simulink model "manipulator_identification_q3"  (R2020a)
settings: Solver=VariableStepAuto  StartTime=0.0  StopTime=Ttot  RelTol=1e-3
undefined symbols (not defined in the file): dT_target, Fq_interp, KpPos_3, KpVel_3, Q_interp, Qp_interp, Qpp_interp, smiData, TdPos_3, TdVel_3, TiPos_3, TiVel_3, X, Y, Z
libraries: sm_lib x46, nesl_utility x23
(part 1 of 2)
settings Model: Creator=monti  LastModifiedBy=miche
settings DebuggingCC: SFMachineParentedDataDiag=error

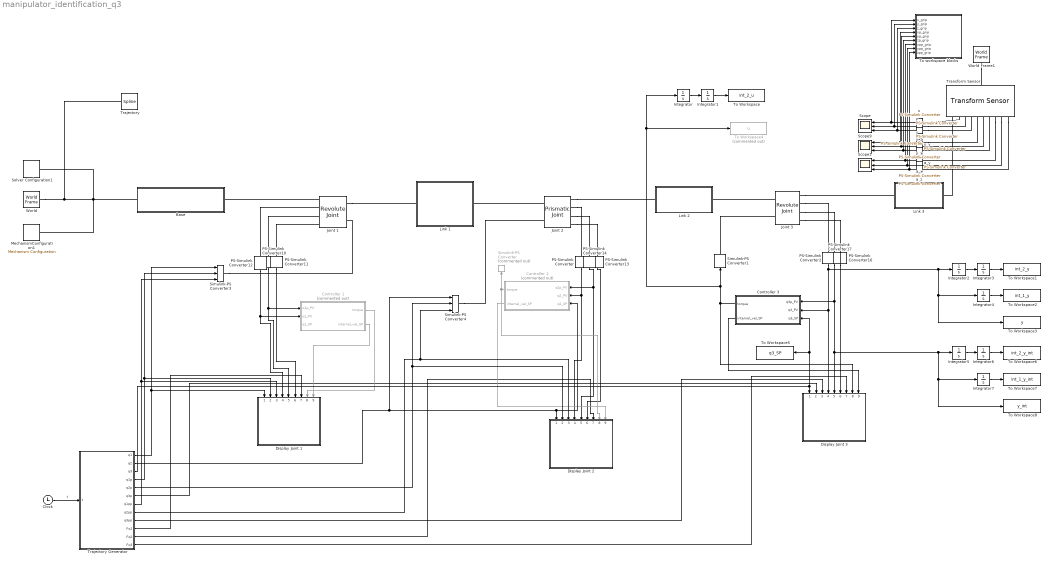
== system manipulator_identification_q3 ==
  Base : Subsystem
      mask Display: image('$imagefile'); % Use "Edit Image" on toolstrip to change.
  Clock : Clock
  Controller 1 : Subsystem  Commented=on
  Controller 2 : Subsystem  Commented=on
  Controller 3 : Subsystem
  Display Joint 1 : Subsystem
  Display Joint 2 : Subsystem
  Display Joint 3 : Subsystem
  Integrator{,1..7} (8 alike) : Integrator
  Joint 1 : sm_lib/Joints/Revolute Joint  JointMode=Normal  SenseConstraintForce=off  SenseConstraintForceX=off  SenseConstraintForceY=off  SenseConstraintForceZ=off  SenseConstraintTorque=off  SenseConstraintTorqueX=off  SenseConstraintTorqueY=off  SenseConstraintTorqueZ=off  SenseTotalForce=off  SenseTotalForceX=off  SenseTotalForceY=off  SenseTotalForceZ=off  SenseTotalTorque=off  SenseTotalTorqueX=off  SenseTotalTorqueY=off  SenseTotalTorqueZ=off  CompositeWrenchDir=FollowerOnBase  CompositeWrenchFrame=BaseFrame  EquilibriumPosition=0  EquilibriumPositionUnits=rad  SpringStiffness=0  SpringStiffnessUnits=N*m/rad  DampingCoefficient=0  DampingCoefficientUnits=N*m/(rad/s)  TorqueActuationMode=ComputedTorque  MotionActuationMode=InputMotion  SensePosition=on  SenseVelocity=on  SenseAcceleration=on  SenseTorqueForce=off  SenseLowerLimitTorqueForce=off  SenseUpperLimitTorqueForce=off  LowerLimitSpecify=on  LowerLimitBound=-180  LowerLimitBoundUnits=deg  LowerLimitStiffness=1e4  LowerLimitStiffnessUnits=N*m/deg  LowerLimitDamping=10  LowerLimitDampingUnits=N*m/(deg/s)  LowerLimitTransitionRegionWidth=0.1  LowerLimitTransitionRegionWidthUnits=deg  UpperLimitSpecify=on  UpperLimitBound=180  UpperLimitBoundUnits=deg  UpperLimitStiffness=1e4  UpperLimitStiffnessUnits=N*m/deg  UpperLimitDamping=10  UpperLimitDampingUnits=N*m/(deg/s)  UpperLimitTransitionRegionWidth=0.1  UpperLimitTransitionRegionWidthUnits=deg  PositionTargetSpecify=on  PositionTargetPriority=Low  PositionTargetValue=0  PositionTargetValueUnits=deg  VelocityTargetSpecify=off  VelocityTargetPriority=High  VelocityTargetValue=0  VelocityTargetValueUnits=deg/s
  Joint 2 : sm_lib/Joints/Prismatic Joint  JointMode=Normal  SenseConstraintForce=off  SenseConstraintForceX=off  SenseConstraintForceY=off  SenseConstraintForceZ=off  SenseConstraintTorque=off  SenseConstraintTorqueX=off  SenseConstraintTorqueY=off  SenseConstraintTorqueZ=off  SenseTotalForce=off  SenseTotalForceX=off  SenseTotalForceY=off  SenseTotalForceZ=off  SenseTotalTorque=off  SenseTotalTorqueX=off  SenseTotalTorqueY=off  SenseTotalTorqueZ=off  CompositeWrenchDir=FollowerOnBase  CompositeWrenchFrame=BaseFrame  EquilibriumPosition=0  EquilibriumPositionUnits=m  SpringStiffness=0  SpringStiffnessUnits=N/m  DampingCoefficient=0  DampingCoefficientUnits=N/(m/s)  TorqueActuationMode=ComputedTorque  MotionActuationMode=InputMotion  SensePosition=on  SenseVelocity=on  SenseAcceleration=on  SenseTorqueForce=off  SenseLowerLimitTorqueForce=off  SenseUpperLimitTorqueForce=off  LowerLimitSpecify=on  LowerLimitBound=0  LowerLimitBoundUnits=m  LowerLimitStiffness=1e6  LowerLimitStiffnessUnits=N/m  LowerLimitDamping=1e3  LowerLimitDampingUnits=N/(m/s)  LowerLimitTransitionRegionWidth=1e-4  LowerLimitTransitionRegionWidthUnits=m  UpperLimitSpecify=on  UpperLimitBound=0.4  UpperLimitBoundUnits=m  UpperLimitStiffness=1e6  UpperLimitStiffnessUnits=N/m  UpperLimitDamping=1e3  UpperLimitDampingUnits=N/(m/s)  UpperLimitTransitionRegionWidth=1e-4  UpperLimitTransitionRegionWidthUnits=m  PositionTargetSpecify=on  PositionTargetPriority=Low  PositionTargetValue=0.000  PositionTargetValueUnits=m  VelocityTargetSpecify=off  VelocityTargetPriority=High  VelocityTargetValue=0  VelocityTargetValueUnits=m/s
  Joint 3 : sm_lib/Joints/Revolute Joint  JointMode=Normal  SenseConstraintForce=off  SenseConstraintForceX=off  SenseConstraintForceY=off  SenseConstraintForceZ=off  SenseConstraintTorque=off  SenseConstraintTorqueX=off  SenseConstraintTorqueY=off  SenseConstraintTorqueZ=off  SenseTotalForce=off  SenseTotalForceX=off  SenseTotalForceY=off  SenseTotalForceZ=off  SenseTotalTorque=off  SenseTotalTorqueX=off  SenseTotalTorqueY=off  SenseTotalTorqueZ=off  CompositeWrenchDir=FollowerOnBase  CompositeWrenchFrame=BaseFrame  EquilibriumPosition=0  EquilibriumPositionUnits=rad  SpringStiffness=0  SpringStiffnessUnits=N*m/rad  DampingCoefficient=0  DampingCoefficientUnits=N*m/(rad/s)  TorqueActuationMode=InputTorque  MotionActuationMode=ComputedMotion  SensePosition=on  SenseVelocity=on  SenseAcceleration=on  SenseTorqueForce=off  SenseLowerLimitTorqueForce=off  SenseUpperLimitTorqueForce=off  LowerLimitSpecify=on  LowerLimitBound=-90  LowerLimitBoundUnits=deg  LowerLimitStiffness=1e4  LowerLimitStiffnessUnits=N*m/deg  LowerLimitDamping=10  LowerLimitDampingUnits=N*m/(deg/s)  LowerLimitTransitionRegionWidth=0.1  LowerLimitTransitionRegionWidthUnits=deg  UpperLimitSpecify=on  UpperLimitBound=90  UpperLimitBoundUnits=deg  UpperLimitStiffness=1e4  UpperLimitStiffnessUnits=N*m/deg  UpperLimitDamping=10  UpperLimitDampingUnits=N*m/(deg/s)  UpperLimitTransitionRegionWidth=0.1  UpperLimitTransitionRegionWidthUnits=deg  PositionTargetSpecify=on  PositionTargetPriority=Low  PositionTargetValue=0  PositionTargetValueUnits=deg  VelocityTargetSpecify=off  VelocityTargetPriority=High  VelocityTargetValue=0  VelocityTargetValueUnits=deg/s
  Link 1 : Subsystem
      mask Display: image('$imagefile'); % Use "Edit Image" on toolstrip to change.
  Link 2 : Subsystem
      mask Display: image('$imagefile'); % Use "Edit Image" on toolstrip to change.
  Link 3 : Subsystem
      mask Display: image('$imagefile'); % Use "Edit Image" on toolstrip to change.
  MechanismConfiguration1 : sm_lib/Utilities/Mechanism Configuration  UniformGravity=Constant  GravityVector=[0 0 -9.80665]  GravityUnits=m/s^2  LinearizationDelta=0.001
  PS-Simulink Converter : nesl_utility/PS-Simulink Converter  PhysicalDomain=network_engine_domain  SubClassName=ps_output  LeftPortType=input  RightPortType=output  PseudoPeriodic=off  Frequencies=[]  Unit=m  AffineConversion=off
      settings: SourceProductBaseCode=PW,SS
  PS-Simulink Converter10 : nesl_utility/PS-Simulink Converter  PhysicalDomain=network_engine_domain  SubClassName=ps_output  LeftPortType=input  RightPortType=output  PseudoPeriodic=off  Frequencies=[]  Unit=rad/s  AffineConversion=off
      settings: SourceProductBaseCode=PW,SS
  PS-Simulink Converter11 : nesl_utility/PS-Simulink Converter  PhysicalDomain=network_engine_domain  SubClassName=ps_output  LeftPortType=input  RightPortType=output  PseudoPeriodic=off  Frequencies=[]  Unit=rad/s^2  AffineConversion=off
      settings: SourceProductBaseCode=PW,SS
  PS-Simulink Converter12 : nesl_utility/PS-Simulink Converter  PhysicalDomain=network_engine_domain  SubClassName=ps_output  LeftPortType=input  RightPortType=output  PseudoPeriodic=off  Frequencies=[]  Unit=rad  AffineConversion=off
      settings: SourceProductBaseCode=PW,SS
  PS-Simulink Converter13 : nesl_utility/PS-Simulink Converter  PhysicalDomain=network_engine_domain  SubClassName=ps_output  LeftPortType=input  RightPortType=output  PseudoPeriodic=off  Frequencies=[]  Unit=m/s^2  AffineConversion=off
      settings: SourceProductBaseCode=PW,SS
  PS-Simulink Converter14 : nesl_utility/PS-Simulink Converter  PhysicalDomain=network_engine_domain  SubClassName=ps_output  LeftPortType=input  RightPortType=output  PseudoPeriodic=off  Frequencies=[]  Unit=m/s  AffineConversion=off
      settings: SourceProductBaseCode=PW,SS
  PS-Simulink Converter16 : nesl_utility/PS-Simulink Converter  PhysicalDomain=network_engine_domain  SubClassName=ps_output  LeftPortType=input  RightPortType=output  PseudoPeriodic=off  Frequencies=[]  Unit=rad/s^2  AffineConversion=off
      settings: SourceProductBaseCode=PW,SS
  PS-Simulink Converter17 : nesl_utility/PS-Simulink Converter  PhysicalDomain=network_engine_domain  SubClassName=ps_output  LeftPortType=input  RightPortType=output  PseudoPeriodic=off  Frequencies=[]  Unit=rad/s  AffineConversion=off
      settings: SourceProductBaseCode=PW,SS
  PS-Simulink Converter2 : nesl_utility/PS-Simulink Converter  PhysicalDomain=network_engine_domain  SubClassName=ps_output  LeftPortType=input  RightPortType=output  PseudoPeriodic=off  Frequencies=[]  Unit=rad  AffineConversion=off
      settings: SourceProductBaseCode=PW,SS
  Scope : Scope  NumInputPorts=3
  Scope1 : Scope  NumInputPorts=3
  Scope9 : Scope  NumInputPorts=3
  Simulink-PS Converter : nesl_utility/Simulink-PS Converter  Commented=on  PhysicalDomain=network_engine_domain  SubClassName=ps_input  LeftPortType=input  RightPortType=output  PseudoPeriodic=off  Frequencies=[]  NoiseDistribution=none  NoiseParameters=[]  Unit=N  AffineConversion=off  FilteringAndDerivatives=provide  SimscapeFilterOrder=1  InputFilterTimeConstant=0.001  UdotUserProvided=0
  Simulink-PS Converter1 : nesl_utility/Simulink-PS Converter  PhysicalDomain=network_engine_domain  SubClassName=ps_input  LeftPortType=input  RightPortType=output  PseudoPeriodic=off  Frequencies=[]  NoiseDistribution=none  NoiseParameters=[]  Unit=N*m  AffineConversion=off  FilteringAndDerivatives=provide  SimscapeFilterOrder=1  InputFilterTimeConstant=0.001  UdotUserProvided=0
  Simulink-PS Converter3 : nesl_utility/Simulink-PS Converter  PhysicalDomain=network_engine_domain  SubClassName=ps_input  LeftPortType=input  RightPortType=output  PseudoPeriodic=off  Frequencies=[]  NoiseDistribution=none  NoiseParameters=[]  Unit=rad  AffineConversion=off  FilteringAndDerivatives=provide  SimscapeFilterOrder=2  InputFilterTimeConstant=0.001  UdotUserProvided=2
      settings: SourceProductBaseCode=PW,SS
  Simulink-PS Converter4 : nesl_utility/Simulink-PS Converter  PhysicalDomain=network_engine_domain  SubClassName=ps_input  LeftPortType=input  RightPortType=output  PseudoPeriodic=off  Frequencies=[]  NoiseDistribution=none  NoiseParameters=[]  Unit=m  AffineConversion=off  FilteringAndDerivatives=provide  SimscapeFilterOrder=2  InputFilterTimeConstant=0.001  UdotUserProvided=2
      settings: SourceProductBaseCode=PW,SS
  Solver Configuration1 : nesl_utility/Solver Configuration  PhysicalDomain=network_engine_domain  SubClassName=solver  LeftPortType=input  RightPortType=generic  Tones=[]  Harmonics=[]  SimulateNoise=off  Profile=off  UseLocalSampling=off  EnableSwitchedLinearOptims=on  FrequencyDomain=off  UseCCode=off  RelTol=0.001  AbsTol=1e-06  MinStep=1e-09  ToWorkspace=off  RevertToSquareIcSolve=off  NumHomotopyIterations=100  PhasorMode=off  PhasorModeNumHarmonics=1  DoDC=off  ResidualTolerance=1e-09  UseLocalSolver=off  LocalSolverChoice=NE_BACKWARD_EULER_ADVANCER  LocalSolverSampleTime=0.001  DoFixedCost=off  MaxNonlinIter=3  MaxModeIter=2  LinearAlgebra=auto  EquationFormulation=NE_TIME_EF  DelaysMemoryBudget=1024  AutomaticFiltering=on  FilteringTimeConstant=0.001  PartitionStorageMethod=AS_NEEDED  PartitionMemoryBudget=1024  PartitionMethod=ROBUST
      settings: SourceProductBaseCode=PW,SS
  To Workspace : ToWorkspace  VariableName=int_2_u  SaveFormat=Timeseries  SampleTime=-1
  To Workspace1 : ToWorkspace  VariableName=int_2_y  SaveFormat=Timeseries  SampleTime=-1
  To Workspace2 : ToWorkspace  VariableName=int_1_y  SaveFormat=Timeseries  SampleTime=-1
  To Workspace3 : ToWorkspace  VariableName=y  SaveFormat=Timeseries  SampleTime=-1
  To Workspace4 : ToWorkspace  Commented=on  VariableName=u  SaveFormat=Timeseries  SampleTime=-1
  To Workspace5 : ToWorkspace  VariableName=q3_SP  SaveFormat=Timeseries  SampleTime=-1
  To Workspace6 : ToWorkspace  VariableName=int_2_y_int  SaveFormat=Timeseries  SampleTime=-1
  To Workspace7 : ToWorkspace  VariableName=int_1_y_int  SaveFormat=Timeseries  SampleTime=-1
  To Workspace8 : ToWorkspace  VariableName=y_int  SaveFormat=Timeseries  SampleTime=-1
  To workspace blocks : Subsystem
  Trajectory : sm_lib/Curves and Surfaces/Spline  GraphicAmbientColor=[0.15 0.15 0.15 1.0]  GraphicDiffuseColor=[0.0 0.0 0.0]  DataPoints=S(1:3,2:end-1)'  DataPointsUnits=m  GraphicEmissiveColor=[0.0 0.0 0.0 1.0]  EndConditionType=Natural  MarkerShape=Sphere  MarkerSize=10  GraphicType=FromGeometry  GraphicOpacity=1  GraphicShininess=75  GraphicSpecularColor=[0.5 0.5 0.5 1.0]  GraphicVisPropType=SimpleVisualProperties
  Trajectory Generator : MATLAB Function  TreatAsAtomicUnit=on
  Transform Sensor : sm_lib/Frames and Transforms/Transform Sensor  MeasurementFrame=World  SenseAngle=off  SenseAxis=off  SenseAngle1=off  SenseAngle2=off  SenseAngle3=off  SenseQ=off  SenseR=off  SenseOmegaX=off  SenseOmegaY=off  SenseOmegaZ=off  SenseOmega1=off  SenseOmega2=off  SenseOmega3=off  SenseQDot=off  SenseRDot=off  SenseAlphaX=off  SenseAlphaY=off  SenseAlphaZ=off  SenseAlpha1=off  SenseAlpha2=off  SenseAlpha3=off  SenseQDDot=off  SenseRDDot=off  SenseX=on  SenseY=on  SenseZ=on  SenseRad=off  SenseAzim=off  SenseDist=off  SenseInc=off  SenseXDot=on  SenseYDot=on  SenseZDot=on  SenseRadDot=off  SenseAzimDot=off  SenseDistDot=off  SenseIncDot=off  SenseXDDot=on  SenseYDDot=on  SenseZDDot=on  SenseRadDDot=off  SenseAzimDDot=off  SenseDistDDot=off  SenseIncDDot=off
  World : sm_lib/Frames and Transforms/World Frame
  World Frame1 : sm_lib/Frames and Transforms/World Frame
  a_x : nesl_utility/PS-Simulink Converter  PhysicalDomain=network_engine_domain  SubClassName=ps_output  LeftPortType=input  RightPortType=output  PseudoPeriodic=off  Frequencies=[]  Unit=m/s^2  AffineConversion=off
  a_y : nesl_utility/PS-Simulink Converter  PhysicalDomain=network_engine_domain  SubClassName=ps_output  LeftPortType=input  RightPortType=output  PseudoPeriodic=off  Frequencies=[]  Unit=m/s^2  AffineConversion=off
  a_z : nesl_utility/PS-Simulink Converter  PhysicalDomain=network_engine_domain  SubClassName=ps_output  LeftPortType=input  RightPortType=output  PseudoPeriodic=off  Frequencies=[]  Unit=m/s^2  AffineConversion=off
  v_x : nesl_utility/PS-Simulink Converter  PhysicalDomain=network_engine_domain  SubClassName=ps_output  LeftPortType=input  RightPortType=output  PseudoPeriodic=off  Frequencies=[]  Unit=m/s  AffineConversion=off
  v_y : nesl_utility/PS-Simulink Converter  PhysicalDomain=network_engine_domain  SubClassName=ps_output  LeftPortType=input  RightPortType=output  PseudoPeriodic=off  Frequencies=[]  Unit=m/s  AffineConversion=off
  v_z : nesl_utility/PS-Simulink Converter  PhysicalDomain=network_engine_domain  SubClassName=ps_output  LeftPortType=input  RightPortType=output  PseudoPeriodic=off  Frequencies=[]  Unit=m/s  AffineConversion=off
  x : nesl_utility/PS-Simulink Converter  PhysicalDomain=network_engine_domain  SubClassName=ps_output  LeftPortType=input  RightPortType=output  PseudoPeriodic=off  Frequencies=[]  Unit=m  AffineConversion=off
  y : nesl_utility/PS-Simulink Converter  PhysicalDomain=network_engine_domain  SubClassName=ps_output  LeftPortType=input  RightPortType=output  PseudoPeriodic=off  Frequencies=[]  Unit=m  AffineConversion=off
  z : nesl_utility/PS-Simulink Converter  PhysicalDomain=network_engine_domain  SubClassName=ps_output  LeftPortType=input  RightPortType=output  PseudoPeriodic=off  Frequencies=[]  Unit=m  AffineConversion=off
  wires:
  Trajectory Generator/9(q3pp) -> Display Joint 3/3(qpp_SP)
  a_y/1 -> Scope1/2, To workspace blocks/8(ypp_grip)
  Clock/1 -> Trajectory Generator/1(t)  "t"
  z/1 -> Scope/3, To workspace blocks/3(z_grip)
  v_y/1 -> Scope9/2, To workspace blocks/5(yp_grip)
  v_z/1 -> Scope9/3, To workspace blocks/6(zp_grip)
  Trajectory Generator/6(q3p) -> Display Joint 3/2(qp_SP)
  PS-Simulink Converter16/1 -> Display Joint 3/6(qpp_PV)
  PS-Simulink Converter12/1 -> Controller 1/2(q1_PV), Display Joint 1/4(q_PV)
  PS-Simulink Converter10/1 -> Controller 1/1(q1p_PV), Display Joint 1/5(qp_PV)
  Trajectory Generator/11(Fq2) -> Display Joint 2/7(torque_theoric)
  PS-Simulink Converter11/1 -> Display Joint 1/6(qpp_PV)
  PS-Simulink Converter/1 -> Display Joint 2/4(q_PV), Controller 2/2(q2_PV)
  Controller 3/2(internal_vel_SP) -> Display Joint 3/9(internal_vel_SP)
  Trajectory Generator/12(Fq3) -> Display Joint 3/7(torque_theoric)
  Trajectory Generator/7(q1pp) -> Simulink-PS Converter3/3, Display Joint 1/3(qpp_SP)
  a_z/1 -> Scope1/3, To workspace blocks/9(zpp_grip)
  PS-Simulink Converter14/1 -> Display Joint 2/5(qp_PV), Controller 2/1(q2p_PV)
  Trajectory Generator/4(q1p) -> Simulink-PS Converter3/2, Display Joint 1/2(qp_SP)
  x/1 -> Scope/1, To workspace blocks/1(x_grip)
  v_x/1 -> Scope9/1, To workspace blocks/4(xp_grip)
  y/1 -> Scope/2, To workspace blocks/2(y_grip)
  PS-Simulink Converter13/1 -> Display Joint 2/6(qpp_PV)
  a_x/1 -> Scope1/1, To workspace blocks/7(xpp_grip)
  Controller 1/1(torque) -> Display Joint 1/8(torque_actual)
  Controller 1/2(internal_vel_SP) -> Display Joint 1/9(internal_vel_SP)
  Trajectory Generator/10(Fq1) -> Display Joint 1/7(torque_theoric)
  Controller 2/1(torque) -> Display Joint 2/8(torque_actual), Simulink-PS Converter/1
  Controller 2/2(internal_vel_SP) -> Display Joint 2/9(internal_vel_SP)
  Integrator4/1 -> To Workspace2/1
  Integrator2/1 -> Integrator3/1
  Integrator3/1 -> To Workspace1/1
  PS-Simulink Converter2/1 -> To Workspace3/1, Integrator4/1, Integrator2/1, Display Joint 3/4(q_PV), Controller 3/2(q3_PV)
  Integrator/1 -> Integrator1/1
  Integrator1/1 -> To Workspace/1
  Controller 3/1(torque) -> Display Joint 3/8(torque_actual), To Workspace4/1, Integrator/1, Simulink-PS Converter1/1
  Trajectory Generator/1(q1) -> Simulink-PS Converter3/1, Display Joint 1/1(q_SP)
  Trajectory Generator/5(q2p) -> Simulink-PS Converter4/2, Display Joint 2/2(qp_SP)
  Trajectory Generator/8(q2pp) -> Simulink-PS Converter4/3, Display Joint 2/3(qpp_SP)
  Trajectory Generator/2(q2) -> Simulink-PS Converter4/1, Controller 2/3(q2_SP), Display Joint 2/1(q_SP)
  Trajectory Generator/3(q3) -> Display Joint 3/1(q_SP), To Workspace5/1, Controller 3/3(q3_SP)
  Integrator6/1 -> To Workspace6/1
  PS-Simulink Converter17/1 -> To Workspace8/1, Integrator7/1, Integrator5/1, Display Joint 3/5(qp_PV), Controller 3/1(q3p_PV)
  Integrator7/1 -> To Workspace7/1
  Integrator5/1 -> Integrator6/1
  connections:
  MechanismConfiguration1/RConn1 -- World/RConn1 -- Trajectory/LConn1 -- Solver Configuration1/RConn1 -- Base/LConn1
  v_z/LConn1 -- Transform Sensor/RConn7
  Joint 3/LConn1 -- Link 2/RConn1
  Joint 2/RConn1 -- Link 2/LConn1
  Joint 1/RConn2 -- PS-Simulink Converter12/LConn1
  Joint 2/RConn2 -- PS-Simulink Converter/LConn1
  Joint 3/RConn3 -- PS-Simulink Converter17/LConn1
  Joint 1/LConn1 -- Link 1/LConn1
  v_y/LConn1 -- Transform Sensor/RConn6
  v_x/LConn1 -- Transform Sensor/RConn5
  Joint 3/RConn4 -- PS-Simulink Converter16/LConn1
  World Frame1/RConn1 -- Transform Sensor/LConn1
  Transform Sensor/RConn8 -- a_x/LConn1
  Joint 3/LConn2 -- Simulink-PS Converter1/RConn1
  Joint 2/RConn3 -- PS-Simulink Converter14/LConn1
  Joint 1/RConn4 -- PS-Simulink Converter11/LConn1
  z/LConn1 -- Transform Sensor/RConn4
  Joint 2/RConn4 -- PS-Simulink Converter13/LConn1
  Transform Sensor/RConn9 -- a_y/LConn1
  Joint 1/RConn3 -- PS-Simulink Converter10/LConn1
  Joint 3/RConn1 -- Link 3/RConn1
  Joint 2/LConn1 -- Link 1/RConn1
  Joint 3/RConn2 -- PS-Simulink Converter2/LConn1
  y/LConn1 -- Transform Sensor/RConn3
  Transform Sensor/RConn10 -- a_z/LConn1
  Joint 1/RConn1 -- Base/RConn1
  x/LConn1 -- Transform Sensor/RConn2
  Transform Sensor/RConn1 -- Link 3/LConn1
  Simulink-PS Converter3/RConn1 -- Joint 1/LConn2
  Simulink-PS Converter4/RConn1 -- Joint 2/LConn2

== system manipulator_identification_q3/Base ==
  Transform : sm_lib/Frames and Transforms/Rigid Transform  TranslationMethod=Cartesian  TranslationStandardOffset=0  TranslationLengthUnit=mm  TranslationStandardAxis=+Z  TranslationCartesianOffset=smiData.RigidTransform(17).translation  TranslationROffset=0  TranslationROffsetUnits=m  TranslationZOffset=0  TranslationZOffsetUnits=m  TranslationThetaOffset=0  TranslationThetaOffsetUnits=deg  RotationMethod=ArbitraryAxis  RotationAngleUnits=rad  RotationStandardAxis=+Z  RotationAngle=smiData.RigidTransform(17).angle  RotationArbitraryAxis=smiData.RigidTransform(17).axis  FollAlignAxisA=+X  BaseAlignAxisA=+Y  FollAlignAxisB=+Y  BaseAlignAxisB=+Z  RotationSequenceAxes=FollowerAxes  RotationSequence=XYX  RotationSequenceAngles=[0 0 0]  RotationSequenceAnglesUnits=deg  RotationMatrix=[1 0 0; 0 1 0; 0 0 1]
  base_2_RIGID : Subsystem
  F1 : PMIOPort  Side=Left
  F : PMIOPort  Port=2  Side=Right
  connections:
  Transform/RConn1 -- base_2_RIGID/LConn1
  F/RConn1 -- base_2_RIGID/RConn1
  F1/RConn1 -- Transform/LConn1

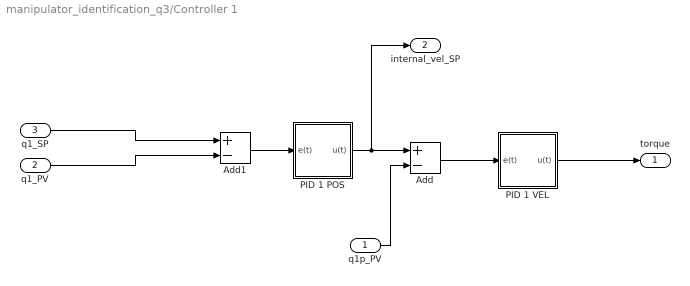
== system manipulator_identification_q3/Controller 1 ==
  q1p_PV : Inport
  q1_PV : Inport  Port=2
  q1_SP : Inport  Port=3
  Add : Sum  Inputs=+-
  Add1 : Sum  Inputs=+-
  PID 1 POS : Subsystem  mask(PID){Kp=1, Ti=0.8, Td=0}
      mask help: Standard formulation
  PID 1 VEL : Subsystem  mask(PID){Kp=10, Ti=0.05, Td=0}
      mask help: Standard formulation
  torque : Outport
  internal_vel_SP : Outport  Port=2
  wires:
  q1_PV/1 -> Add1/2
  Add1/1 -> PID 1 POS/1(e(t))
  Add/1 -> PID 1 VEL/1(e(t))
  PID 1 POS/1(u(t)) -> internal_vel_SP/1, Add/1
  PID 1 VEL/1(u(t)) -> torque/1
  q1p_PV/1 -> Add/2
  q1_SP/1 -> Add1/1

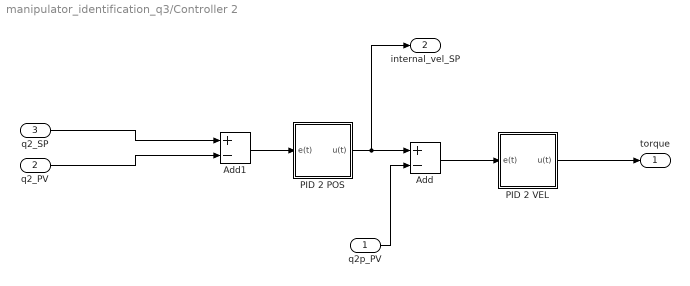
== system manipulator_identification_q3/Controller 2 ==
  q2p_PV : Inport
  q2_PV : Inport  Port=2
  q2_SP : Inport  Port=3
  Add : Sum  Inputs=+-
  Add1 : Sum  Inputs=+-
  PID 2 POS : Subsystem  mask(PID){Kp=100, Ti=0.01, Td=0}
      mask help: Standard formulation
  PID 2 VEL : Subsystem  mask(PID){Kp=10, Ti=10, Td=1}
      mask help: Standard formulation
  torque : Outport
  internal_vel_SP : Outport  Port=2
  wires:
  q2_PV/1 -> Add1/2
  Add1/1 -> PID 2 POS/1(e(t))
  Add/1 -> PID 2 VEL/1(e(t))
  PID 2 POS/1(u(t)) -> internal_vel_SP/1, Add/1
  PID 2 VEL/1(u(t)) -> torque/1
  q2p_PV/1 -> Add/2
  q2_SP/1 -> Add1/1

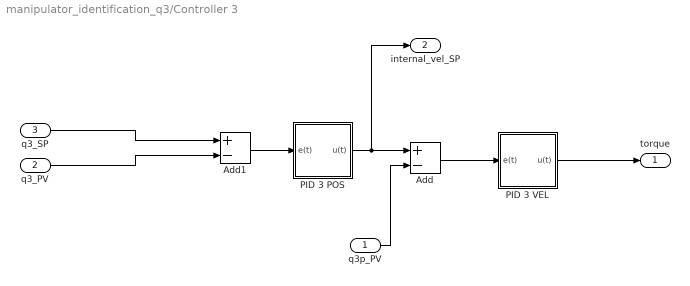
== system manipulator_identification_q3/Controller 3 ==
  q3p_PV : Inport
  q3_PV : Inport  Port=2
  q3_SP : Inport  Port=3
  Add : Sum  Inputs=+-
  Add1 : Sum  Inputs=+-
  PID 3 POS : Subsystem  mask(PID){Kp=KpPos_3, Ti=TiPos_3, Td=TdPos_3}
      mask help: Standard formulation
  PID 3 VEL : Subsystem  mask(PID){Kp=KpVel_3, Ti=TiVel_3, Td=TdVel_3}
      mask help: Standard formulation
  torque : Outport
  internal_vel_SP : Outport  Port=2
  wires:
  q3_PV/1 -> Add1/2
  Add1/1 -> PID 3 POS/1(e(t))
  Add/1 -> PID 3 VEL/1(e(t))
  PID 3 POS/1(u(t)) -> internal_vel_SP/1, Add/1
  PID 3 VEL/1(u(t)) -> torque/1
  q3p_PV/1 -> Add/2
  q3_SP/1 -> Add1/1

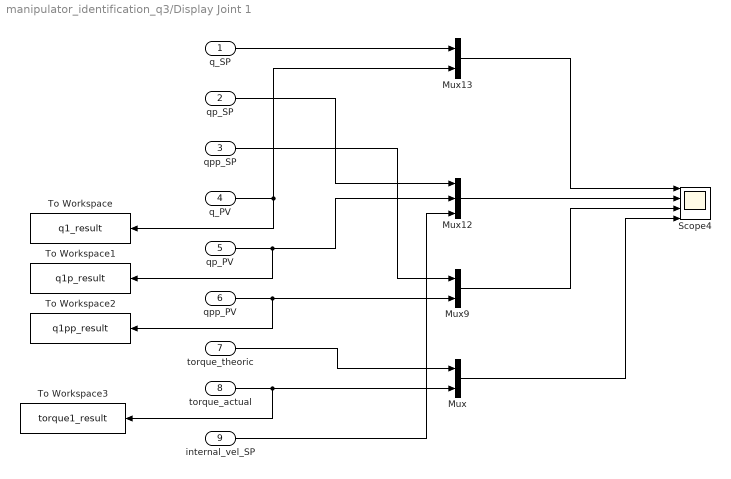
== system manipulator_identification_q3/Display Joint 1 ==
  q_SP : Inport
  qp_SP : Inport  Port=2
  qpp_SP : Inport  Port=3
  q_PV : Inport  Port=4
  qp_PV : Inport  Port=5
  qpp_PV : Inport  Port=6
  torque_theoric : Inport  Port=7
  torque_actual : Inport  Port=8
  internal_vel_SP : Inport  Port=9
  Mux : Mux  Inputs=2
  Mux12 : Mux  Inputs=3
  Mux13 : Mux  Inputs=2
  Mux9 : Mux  Inputs=2
  Scope4 : Scope  NumInputPorts=4
  To Workspace : ToWorkspace  VariableName=q1_result  SaveFormat=Timeseries  SampleTime=-1
  To Workspace1 : ToWorkspace  VariableName=q1p_result  SaveFormat=Timeseries  SampleTime=-1
  To Workspace2 : ToWorkspace  VariableName=q1pp_result  SaveFormat=Timeseries  SampleTime=-1
  To Workspace3 : ToWorkspace  VariableName=torque1_result  SaveFormat=Timeseries  SampleTime=-1
  wires:
  q_SP/1 -> Mux13/1
  qp_SP/1 -> Mux12/1
  qpp_SP/1 -> Mux9/1
  Mux12/1 -> Scope4/2
  Mux13/1 -> Scope4/1
  Mux9/1 -> Scope4/3
  torque_actual/1 -> Mux/2, To Workspace3/1
  q_PV/1 -> To Workspace/1, Mux13/2
  qp_PV/1 -> To Workspace1/1, Mux12/2
  qpp_PV/1 -> To Workspace2/1, Mux9/2
  internal_vel_SP/1 -> Mux12/3
  torque_theoric/1 -> Mux/1
  Mux/1 -> Scope4/4

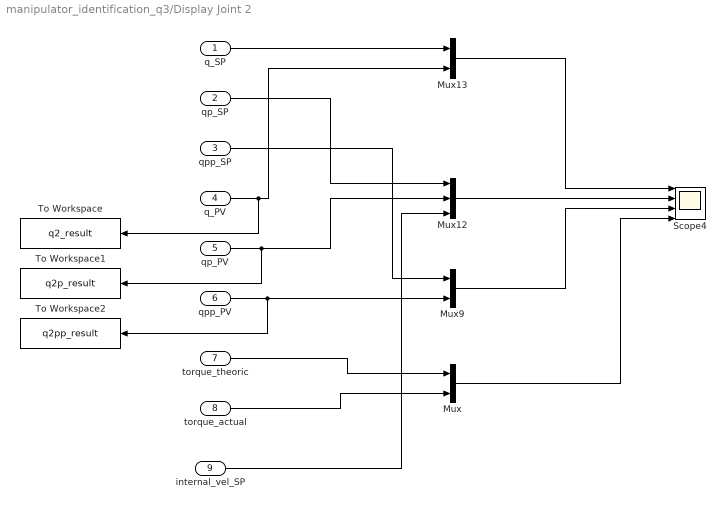
== system manipulator_identification_q3/Display Joint 2 ==
  q_SP : Inport
  qp_SP : Inport  Port=2
  qpp_SP : Inport  Port=3
  q_PV : Inport  Port=4
  qp_PV : Inport  Port=5
  qpp_PV : Inport  Port=6
  torque_theoric : Inport  Port=7
  torque_actual : Inport  Port=8
  internal_vel_SP : Inport  Port=9
  Mux : Mux  Inputs=2
  Mux12 : Mux  Inputs=3
  Mux13 : Mux  Inputs=2
  Mux9 : Mux  Inputs=2
  Scope4 : Scope  NumInputPorts=4
  To Workspace : ToWorkspace  VariableName=q2_result  SaveFormat=Timeseries  SampleTime=-1
  To Workspace1 : ToWorkspace  VariableName=q2p_result  SaveFormat=Timeseries  SampleTime=-1
  To Workspace2 : ToWorkspace  VariableName=q2pp_result  SaveFormat=Timeseries  SampleTime=-1
  wires:
  q_SP/1 -> Mux13/1
  qp_SP/1 -> Mux12/1
  qpp_SP/1 -> Mux9/1
  Mux12/1 -> Scope4/2
  Mux13/1 -> Scope4/1
  Mux9/1 -> Scope4/3
  q_PV/1 -> To Workspace/1, Mux13/2
  qp_PV/1 -> To Workspace1/1, Mux12/2
  qpp_PV/1 -> To Workspace2/1, Mux9/2
  internal_vel_SP/1 -> Mux12/3
  torque_theoric/1 -> Mux/1
  torque_actual/1 -> Mux/2
  Mux/1 -> Scope4/4

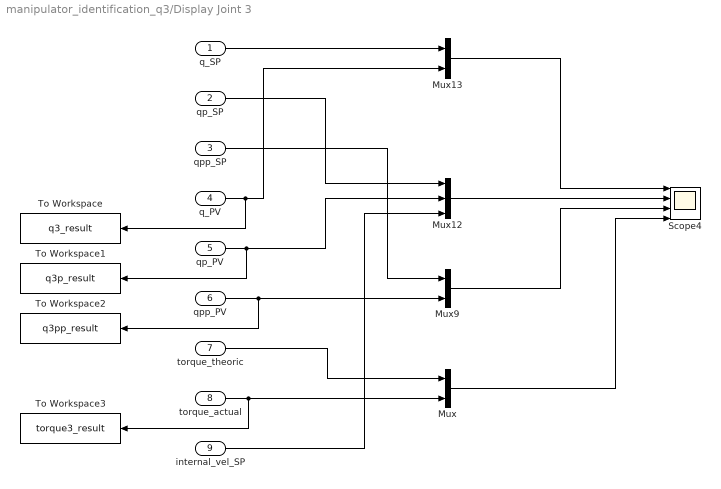
== system manipulator_identification_q3/Display Joint 3 ==
  q_SP : Inport
  qp_SP : Inport  Port=2
  qpp_SP : Inport  Port=3
  q_PV : Inport  Port=4
  qp_PV : Inport  Port=5
  qpp_PV : Inport  Port=6
  torque_theoric : Inport  Port=7
  torque_actual : Inport  Port=8
  internal_vel_SP : Inport  Port=9
  Mux : Mux  Inputs=2
  Mux12 : Mux  Inputs=3
  Mux13 : Mux  Inputs=2
  Mux9 : Mux  Inputs=2
  Scope4 : Scope  NumInputPorts=4
  To Workspace : ToWorkspace  VariableName=q3_result  SaveFormat=Timeseries  SampleTime=-1
  To Workspace1 : ToWorkspace  VariableName=q3p_result  SaveFormat=Timeseries  SampleTime=-1
  To Workspace2 : ToWorkspace  VariableName=q3pp_result  SaveFormat=Timeseries  SampleTime=-1
  To Workspace3 : ToWorkspace  VariableName=torque3_result  SaveFormat=Timeseries  SampleTime=-1
  wires:
  q_SP/1 -> Mux13/1
  q_PV/1 -> To Workspace/1, Mux13/2
  qp_SP/1 -> Mux12/1
  qp_PV/1 -> To Workspace1/1, Mux12/2
  qpp_SP/1 -> Mux9/1
  qpp_PV/1 -> To Workspace2/1, Mux9/2
  Mux12/1 -> Scope4/2
  Mux13/1 -> Scope4/1
  Mux9/1 -> Scope4/3
  torque_actual/1 -> To Workspace3/1, Mux/2
  torque_theoric/1 -> Mux/1
  Mux/1 -> Scope4/4
  internal_vel_SP/1 -> Mux12/3

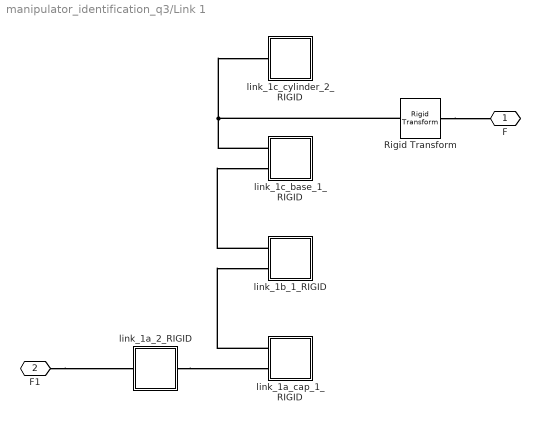
== system manipulator_identification_q3/Link 1 ==
  Rigid Transform : sm_lib/Frames and Transforms/Rigid Transform  TranslationMethod=StandardAxis  TranslationStandardOffset=0.11  TranslationLengthUnit=m  TranslationStandardAxis=+Z  TranslationCartesianOffset=[0 0 0]  TranslationROffset=0  TranslationROffsetUnits=m  TranslationZOffset=0  TranslationZOffsetUnits=m  TranslationThetaOffset=0  TranslationThetaOffsetUnits=deg  RotationMethod=None  RotationAngleUnits=deg  RotationStandardAxis=+Y  RotationAngle=180  RotationArbitraryAxis=[0 0 1]  FollAlignAxisA=+X  BaseAlignAxisA=+Y  FollAlignAxisB=+Y  BaseAlignAxisB=+Z  RotationSequenceAxes=FollowerAxes  RotationSequence=XYX  RotationSequenceAngles=[0 0 0]  RotationSequenceAnglesUnits=deg  RotationMatrix=[1 0 0; 0 1 0; 0 0 1]
  link_1a_2_RIGID : Subsystem
  link_1a_cap_1_RIGID : Subsystem
  link_1b_1_RIGID : Subsystem
  link_1c_base_1_RIGID : Subsystem
  link_1c_cylinder_2_RIGID : Subsystem
  F : PMIOPort  Side=Right
  F1 : PMIOPort  Port=2  Side=Left
  connections:
  link_1c_base_1_RIGID/LConn1 -- Rigid Transform/LConn1 -- link_1c_cylinder_2_RIGID/LConn1
  link_1a_2_RIGID/LConn1 -- link_1a_cap_1_RIGID/LConn2
  link_1b_1_RIGID/LConn1 -- link_1c_base_1_RIGID/LConn2
  F1/RConn1 -- link_1a_2_RIGID/RConn1
  link_1a_cap_1_RIGID/LConn1 -- link_1b_1_RIGID/LConn2
  Rigid Transform/RConn1 -- F/RConn1

== system manipulator_identification_q3/Link 2 ==
  Rigid Transform : sm_lib/Frames and Transforms/Rigid Transform  TranslationMethod=None  TranslationStandardOffset=0  TranslationLengthUnit=m  TranslationStandardAxis=+Z  TranslationCartesianOffset=[0 0 0]  TranslationROffset=0  TranslationROffsetUnits=m  TranslationZOffset=0  TranslationZOffsetUnits=m  TranslationThetaOffset=0  TranslationThetaOffsetUnits=deg  RotationMethod=StandardAxis  RotationAngleUnits=deg  RotationStandardAxis=+X  RotationAngle=180  RotationArbitraryAxis=[0 0 1]  FollAlignAxisA=+X  BaseAlignAxisA=+Y  FollAlignAxisB=+Y  BaseAlignAxisB=+Z  RotationSequenceAxes=FollowerAxes  RotationSequence=XYX  RotationSequenceAngles=[0 0 0]  RotationSequenceAnglesUnits=deg  RotationMatrix=[1 0 0; 0 1 0; 0 0 1]
  Rigid Transform1 : sm_lib/Frames and Transforms/Rigid Transform  TranslationMethod=StandardAxis  TranslationStandardOffset=0.07  TranslationLengthUnit=m  TranslationStandardAxis=+Z  TranslationCartesianOffset=[0 0 0]  TranslationROffset=0  TranslationROffsetUnits=m  TranslationZOffset=0  TranslationZOffsetUnits=m  TranslationThetaOffset=0  TranslationThetaOffsetUnits=deg  RotationMethod=StandardAxis  RotationAngleUnits=deg  RotationStandardAxis=+Y  RotationAngle=180  RotationArbitraryAxis=[0 0 1]  FollAlignAxisA=+X  BaseAlignAxisA=+Y  FollAlignAxisB=+Y  BaseAlignAxisB=+Z  RotationSequenceAxes=FollowerAxes  RotationSequence=XYX  RotationSequenceAngles=[0 0 0]  RotationSequenceAnglesUnits=deg  RotationMatrix=[1 0 0; 0 1 0; 0 0 1]
  link_2_ending_1_RIGID : Subsystem
  link_2_piston_1_RIGID : Subsystem
  F1 : PMIOPort  Side=Left
  F : PMIOPort  Port=2  Side=Right
  connections:
  link_2_ending_1_RIGID/LConn1 -- link_2_piston_1_RIGID/LConn2
  F1/RConn1 -- Rigid Transform/LConn1
  Rigid Transform/RConn1 -- link_2_piston_1_RIGID/LConn1
  Rigid Transform1/LConn1 -- link_2_ending_1_RIGID/RConn1
  Rigid Transform1/RConn1 -- F/RConn1

== system manipulator_identification_q3/Link 3 ==
  link_3_1_RIGID : Subsystem
  F : PMIOPort  Side=Right
  F1 : PMIOPort  Port=2  Side=Left
  connections:
  F/RConn1 -- link_3_1_RIGID/LConn1
  link_3_1_RIGID/LConn2 -- F1/RConn1

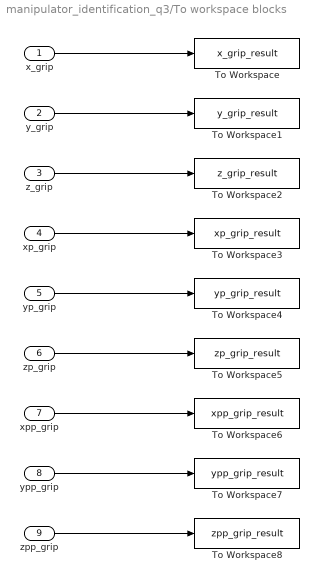
== system manipulator_identification_q3/To workspace blocks ==
  x_grip : Inport
  y_grip : Inport  Port=2
  z_grip : Inport  Port=3
  xp_grip : Inport  Port=4
  yp_grip : Inport  Port=5
  zp_grip : Inport  Port=6
  xpp_grip : Inport  Port=7
  ypp_grip : Inport  Port=8
  zpp_grip : Inport  Port=9
  To Workspace : ToWorkspace  VariableName=x_grip_result  SaveFormat=Timeseries  SampleTime=-1
  To Workspace1 : ToWorkspace  VariableName=y_grip_result  SaveFormat=Timeseries  SampleTime=-1
  To Workspace2 : ToWorkspace  VariableName=z_grip_result  SaveFormat=Timeseries  SampleTime=-1
  To Workspace3 : ToWorkspace  VariableName=xp_grip_result  SaveFormat=Timeseries  SampleTime=-1
  To Workspace4 : ToWorkspace  VariableName=yp_grip_result  SaveFormat=Timeseries  SampleTime=-1
  To Workspace5 : ToWorkspace  VariableName=zp_grip_result  SaveFormat=Timeseries  SampleTime=-1
  To Workspace6 : ToWorkspace  VariableName=xpp_grip_result  SaveFormat=Timeseries  SampleTime=-1
  To Workspace7 : ToWorkspace  VariableName=ypp_grip_result  SaveFormat=Timeseries  SampleTime=-1
  To Workspace8 : ToWorkspace  VariableName=zpp_grip_result  SaveFormat=Timeseries  SampleTime=-1
  wires:
  x_grip/1 -> To Workspace/1
  y_grip/1 -> To Workspace1/1
  z_grip/1 -> To Workspace2/1
  xp_grip/1 -> To Workspace3/1
  zp_grip/1 -> To Workspace5/1
  yp_grip/1 -> To Workspace4/1
  xpp_grip/1 -> To Workspace6/1
  zpp_grip/1 -> To Workspace8/1
  ypp_grip/1 -> To Workspace7/1

== system manipulator_identification_q3/Base/base_2_RIGID ==
  ReferenceFrame : sm_lib/Frames and Transforms/Reference Frame
  Solid : sm_lib/Body Elements/File Solid  ExtGeomFileName=C:\Users\miche\OneDrive - unibs.it\University\Magistrale - UNIBS\1_Primo Anno\Servosystems & Robotics\Servosystems & Robotics Project\Robot Model - Solidworks\Manipulator\simscape_linked_assembly\base_Default_sldprt.STEP  UnitType=FromFile  ExtGeomFileUnits=m  StepReaderType=HEX  ExportConvexHullGeometry=off  InertiaType=Custom  Mass=smiData.Solid(4).mass  MassUnits=kg  CenterOfMass=smiData.Solid(4).CoM  CenterOfMassUnits=mm  MomentsOfInertia=smiData.Solid(4).MoI  MomentsOfInertiaUnits=kg*mm^2  ProductsOfInertia=smiData.Solid(4).PoI  ProductsOfInertiaUnits=kg*mm^2  BasedOnType=DensityFromFile  Density=1000  DensityUnits=kg/m^3  DoExposeReferenceFrame=on  SerializedFrames=<Frames/>  GraphicType=FromGeometry  MarkerShape=Sphere  MarkerSize=10  GraphicVisPropType=SimpleVisualProperties  GraphicDiffuseColor=[1.0 1.0 1.0]  GraphicSpecularColor=[0.5 0.5 0.5 1.0]  GraphicAmbientColor=[0.15 0.15 0.15 1.0]  GraphicEmissiveColor=[0.0 0.0 0.0 1.0]  GraphicShininess=75  GraphicOpacity=smiData.Solid(4).opacity
  Transform : sm_lib/Frames and Transforms/Rigid Transform  TranslationMethod=Cartesian  TranslationStandardOffset=0  TranslationLengthUnit=mm  TranslationStandardAxis=+Z  TranslationCartesianOffset=smiData.RigidTransform(8).translation  TranslationROffset=0  TranslationROffsetUnits=m  TranslationZOffset=0  TranslationZOffsetUnits=m  TranslationThetaOffset=0  TranslationThetaOffsetUnits=deg  RotationMethod=ArbitraryAxis  RotationAngleUnits=rad  RotationStandardAxis=+Z  RotationAngle=smiData.RigidTransform(8).angle  RotationArbitraryAxis=smiData.RigidTransform(8).axis  FollAlignAxisA=+X  BaseAlignAxisA=+Y  FollAlignAxisB=+Y  BaseAlignAxisB=+Z  RotationSequenceAxes=FollowerAxes  RotationSequence=XYX  RotationSequenceAngles=[0 0 0]  RotationSequenceAnglesUnits=deg  RotationMatrix=[1 0 0; 0 1 0; 0 0 1]
  F1 : PMIOPort  Side=Left
  F : PMIOPort  Port=2  Side=Right
  connections:
  Solid/RConn1 -- ReferenceFrame/RConn1 -- Transform/LConn1 -- F1/RConn1
  Transform/RConn1 -- F/RConn1

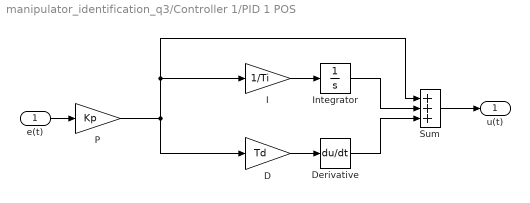
== system manipulator_identification_q3/Controller 1/PID 1 POS ==
  e(t) : Inport
  D : Gain  Gain=Td
  Derivative : Derivative
  I : Gain  Gain=1/Ti
  Integrator : Integrator
  P : Gain  Gain=Kp
  Sum : Sum  Inputs=+++
  u(t) : Outport  VectorParamsAs1DForOutWhenUnconnected=off
  wires:
  P/1 -> I/1, Sum/1, D/1
  I/1 -> Integrator/1
  Integrator/1 -> Sum/2
  D/1 -> Derivative/1
  Derivative/1 -> Sum/3
  Sum/1 -> u(t)/1
  e(t)/1 -> P/1

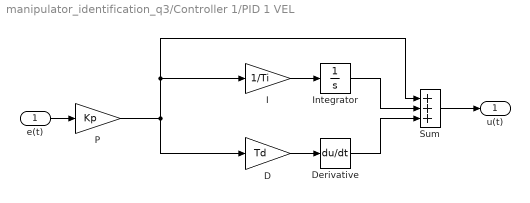
== system manipulator_identification_q3/Controller 1/PID 1 VEL ==
  e(t) : Inport
  D : Gain  Gain=Td
  Derivative : Derivative
  I : Gain  Gain=1/Ti
  Integrator : Integrator
  P : Gain  Gain=Kp
  Sum : Sum  Inputs=+++
  u(t) : Outport  VectorParamsAs1DForOutWhenUnconnected=off
  wires:
  P/1 -> I/1, Sum/1, D/1
  I/1 -> Integrator/1
  Integrator/1 -> Sum/2
  D/1 -> Derivative/1
  Derivative/1 -> Sum/3
  Sum/1 -> u(t)/1
  e(t)/1 -> P/1

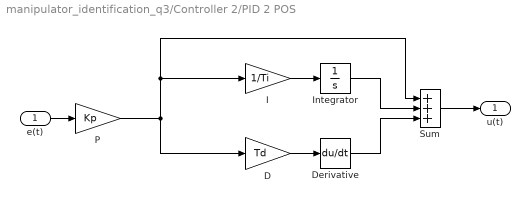
== system manipulator_identification_q3/Controller 2/PID 2 POS ==
  e(t) : Inport
  D : Gain  Gain=Td
  Derivative : Derivative
  I : Gain  Gain=1/Ti
  Integrator : Integrator
  P : Gain  Gain=Kp
  Sum : Sum  Inputs=+++
  u(t) : Outport  VectorParamsAs1DForOutWhenUnconnected=off
  wires:
  P/1 -> I/1, Sum/1, D/1
  I/1 -> Integrator/1
  Integrator/1 -> Sum/2
  D/1 -> Derivative/1
  Derivative/1 -> Sum/3
  Sum/1 -> u(t)/1
  e(t)/1 -> P/1

== system manipulator_identification_q3/Controller 2/PID 2 VEL ==
  e(t) : Inport
  D : Gain  Gain=Td
  Derivative : Derivative
  I : Gain  Gain=1/Ti
  Integrator : Integrator
  P : Gain  Gain=Kp
  Sum : Sum  Inputs=+++
  u(t) : Outport  VectorParamsAs1DForOutWhenUnconnected=off
  wires:
  P/1 -> I/1, Sum/1, D/1
  I/1 -> Integrator/1
  Integrator/1 -> Sum/2
  D/1 -> Derivative/1
  Derivative/1 -> Sum/3
  Sum/1 -> u(t)/1
  e(t)/1 -> P/1

== system manipulator_identification_q3/Controller 3/PID 3 POS ==
  e(t) : Inport
  D : Gain  Gain=Td
  Derivative : Derivative
  I : Gain  Gain=1/Ti
  Integrator : Integrator
  P : Gain  Gain=Kp
  Sum : Sum  Inputs=+++
  u(t) : Outport  VectorParamsAs1DForOutWhenUnconnected=off
  wires:
  P/1 -> I/1, Sum/1, D/1
  I/1 -> Integrator/1
  Integrator/1 -> Sum/2
  D/1 -> Derivative/1
  Derivative/1 -> Sum/3
  Sum/1 -> u(t)/1
  e(t)/1 -> P/1

== system manipulator_identification_q3/Controller 3/PID 3 VEL ==
  e(t) : Inport
  D : Gain  Gain=Td
  Derivative : Derivative
  I : Gain  Gain=1/Ti
  Integrator : Integrator
  P : Gain  Gain=Kp
  Sum : Sum  Inputs=+++
  u(t) : Outport  VectorParamsAs1DForOutWhenUnconnected=off
  wires:
  P/1 -> I/1, Sum/1, D/1
  I/1 -> Integrator/1
  Integrator/1 -> Sum/2
  D/1 -> Derivative/1
  Derivative/1 -> Sum/3
  Sum/1 -> u(t)/1
  e(t)/1 -> P/1

== system manipulator_identification_q3/Link 1/link_1a_2_RIGID ==
  ReferenceFrame : sm_lib/Frames and Transforms/Reference Frame
  Solid : sm_lib/Body Elements/File Solid  ExtGeomFileName=C:\Users\miche\OneDrive - unibs.it\University\Magistrale - UNIBS\1_Primo Anno\Servosystems & Robotics\Servosystems & Robotics Project\Robot Model - Solidworks\Manipulator\simscape_linked_assembly\link_1a_Default_sldprt.STEP  UnitType=FromFile  ExtGeomFileUnits=m  StepReaderType=HEX  ExportConvexHullGeometry=off  InertiaType=Custom  Mass=smiData.Solid(8).mass  MassUnits=kg  CenterOfMass=smiData.Solid(8).CoM  CenterOfMassUnits=cm  MomentsOfInertia=smiData.Solid(8).MoI  MomentsOfInertiaUnits=kg*cm^2  ProductsOfInertia=smiData.Solid(8).PoI  ProductsOfInertiaUnits=kg*cm^2  BasedOnType=DensityFromFile  Density=1000  DensityUnits=kg/m^3  DoExposeReferenceFrame=on  SerializedFrames=<Frames/>  GraphicType=FromGeometry  MarkerShape=Sphere  MarkerSize=10  GraphicVisPropType=SimpleVisualProperties  GraphicDiffuseColor=[1.0 0.4 0.4]  GraphicSpecularColor=[0.5 0.5 0.5 1.0]  GraphicAmbientColor=[0.15 0.15 0.15 1.0]  GraphicEmissiveColor=[0.0 0.0 0.0 1.0]  GraphicShininess=75  GraphicOpacity=smiData.Solid(8).opacity
  Transform : sm_lib/Frames and Transforms/Rigid Transform  TranslationMethod=Cartesian  TranslationStandardOffset=0  TranslationLengthUnit=mm  TranslationStandardAxis=+Z  TranslationCartesianOffset=smiData.RigidTransform(4).translation  TranslationROffset=0  TranslationROffsetUnits=m  TranslationZOffset=0  TranslationZOffsetUnits=m  TranslationThetaOffset=0  TranslationThetaOffsetUnits=deg  RotationMethod=ArbitraryAxis  RotationAngleUnits=rad  RotationStandardAxis=+Z  RotationAngle=smiData.RigidTransform(4).angle  RotationArbitraryAxis=smiData.RigidTransform(4).axis  FollAlignAxisA=+X  BaseAlignAxisA=+Y  FollAlignAxisB=+Y  BaseAlignAxisB=+Z  RotationSequenceAxes=FollowerAxes  RotationSequence=XYX  RotationSequenceAngles=[0 0 0]  RotationSequenceAnglesUnits=deg  RotationMatrix=[1 0 0; 0 1 0; 0 0 1]
  Transform1 : sm_lib/Frames and Transforms/Rigid Transform  TranslationMethod=Cartesian  TranslationStandardOffset=0  TranslationLengthUnit=mm  TranslationStandardAxis=+Z  TranslationCartesianOffset=smiData.RigidTransform(7).translation  TranslationROffset=0  TranslationROffsetUnits=m  TranslationZOffset=0  TranslationZOffsetUnits=m  TranslationThetaOffset=0  TranslationThetaOffsetUnits=deg  RotationMethod=ArbitraryAxis  RotationAngleUnits=rad  RotationStandardAxis=+Z  RotationAngle=smiData.RigidTransform(7).angle  RotationArbitraryAxis=smiData.RigidTransform(7).axis  FollAlignAxisA=+X  BaseAlignAxisA=+Y  FollAlignAxisB=+Y  BaseAlignAxisB=+Z  RotationSequenceAxes=FollowerAxes  RotationSequence=XYX  RotationSequenceAngles=[0 0 0]  RotationSequenceAnglesUnits=deg  RotationMatrix=[1 0 0; 0 1 0; 0 0 1]
  F : PMIOPort  Side=Left
  F1 : PMIOPort  Port=2  Side=Right
  connections:
  Solid/RConn1 -- ReferenceFrame/RConn1 -- Transform/LConn1 -- Transform1/LConn1
  Transform/RConn1 -- F/RConn1
  Transform1/RConn1 -- F1/RConn1

== system manipulator_identification_q3/Link 1/link_1a_cap_1_RIGID ==
  ReferenceFrame : sm_lib/Frames and Transforms/Reference Frame
  Solid : sm_lib/Body Elements/File Solid  ExtGeomFileName=C:\Users\miche\OneDrive - unibs.it\University\Magistrale - UNIBS\1_Primo Anno\Servosystems & Robotics\Servosystems & Robotics Project\Robot Model - Solidworks\Manipulator\simscape_linked_assembly\link_1a_cap_Default_sldprt.STEP  UnitType=FromFile  ExtGeomFileUnits=m  StepReaderType=HEX  ExportConvexHullGeometry=off  InertiaType=Custom  Mass=smiData.Solid(6).mass  MassUnits=kg  CenterOfMass=smiData.Solid(6).CoM  CenterOfMassUnits=cm  MomentsOfInertia=smiData.Solid(6).MoI  MomentsOfInertiaUnits=kg*cm^2  ProductsOfInertia=smiData.Solid(6).PoI  ProductsOfInertiaUnits=kg*cm^2  BasedOnType=DensityFromFile  Density=1000  DensityUnits=kg/m^3  DoExposeReferenceFrame=on  SerializedFrames=<Frames/>  GraphicType=FromGeometry  MarkerShape=Sphere  MarkerSize=10  GraphicVisPropType=SimpleVisualProperties  GraphicDiffuseColor=[1.0 0.4 0.4]  GraphicSpecularColor=[0.5 0.5 0.5 1.0]  GraphicAmbientColor=[0.15 0.15 0.15 1.0]  GraphicEmissiveColor=[0.0 0.0 0.0 1.0]  GraphicShininess=75  GraphicOpacity=smiData.Solid(6).opacity
  Transform : sm_lib/Frames and Transforms/Rigid Transform  TranslationMethod=Cartesian  TranslationStandardOffset=0  TranslationLengthUnit=mm  TranslationStandardAxis=+Z  TranslationCartesianOffset=smiData.RigidTransform(3).translation  TranslationROffset=0  TranslationROffsetUnits=m  TranslationZOffset=0  TranslationZOffsetUnits=m  TranslationThetaOffset=0  TranslationThetaOffsetUnits=deg  RotationMethod=ArbitraryAxis  RotationAngleUnits=rad  RotationStandardAxis=+Z  RotationAngle=smiData.RigidTransform(3).angle  RotationArbitraryAxis=smiData.RigidTransform(3).axis  FollAlignAxisA=+X  BaseAlignAxisA=+Y  FollAlignAxisB=+Y  BaseAlignAxisB=+Z  RotationSequenceAxes=FollowerAxes  RotationSequence=XYX  RotationSequenceAngles=[0 0 0]  RotationSequenceAnglesUnits=deg  RotationMatrix=[1 0 0; 0 1 0; 0 0 1]
  Transform1 : sm_lib/Frames and Transforms/Rigid Transform  TranslationMethod=Cartesian  TranslationStandardOffset=0  TranslationLengthUnit=mm  TranslationStandardAxis=+Z  TranslationCartesianOffset=smiData.RigidTransform(5).translation  TranslationROffset=0  TranslationROffsetUnits=m  TranslationZOffset=0  TranslationZOffsetUnits=m  TranslationThetaOffset=0  TranslationThetaOffsetUnits=deg  RotationMethod=ArbitraryAxis  RotationAngleUnits=rad  RotationStandardAxis=+Z  RotationAngle=smiData.RigidTransform(5).angle  RotationArbitraryAxis=smiData.RigidTransform(5).axis  FollAlignAxisA=+X  BaseAlignAxisA=+Y  FollAlignAxisB=+Y  BaseAlignAxisB=+Z  RotationSequenceAxes=FollowerAxes  RotationSequence=XYX  RotationSequenceAngles=[0 0 0]  RotationSequenceAnglesUnits=deg  RotationMatrix=[1 0 0; 0 1 0; 0 0 1]
  F1 : PMIOPort  Side=Left
  F : PMIOPort  Port=2  Side=Left
  connections:
  Solid/RConn1 -- ReferenceFrame/RConn1 -- Transform/LConn1 -- Transform1/LConn1
  Transform/RConn1 -- F/RConn1
  Transform1/RConn1 -- F1/RConn1

== system manipulator_identification_q3/Link 1/link_1b_1_RIGID ==
  ReferenceFrame : sm_lib/Frames and Transforms/Reference Frame
  Solid : sm_lib/Body Elements/File Solid  ExtGeomFileName=C:\Users\miche\OneDrive - unibs.it\University\Magistrale - UNIBS\1_Primo Anno\Servosystems & Robotics\Servosystems & Robotics Project\Robot Model - Solidworks\Manipulator\simscape_linked_assembly\link_1b_Default_sldprt.STEP  UnitType=FromFile  ExtGeomFileUnits=m  StepReaderType=HEX  ExportConvexHullGeometry=off  InertiaType=Custom  Mass=smiData.Solid(5).mass  MassUnits=kg  CenterOfMass=smiData.Solid(5).CoM  CenterOfMassUnits=cm  MomentsOfInertia=smiData.Solid(5).MoI  MomentsOfInertiaUnits=kg*cm^2  ProductsOfInertia=smiData.Solid(5).PoI  ProductsOfInertiaUnits=kg*cm^2  BasedOnType=DensityFromFile  Density=1000  DensityUnits=kg/m^3  DoExposeReferenceFrame=on  SerializedFrames=<Frames/>  GraphicType=FromGeometry  MarkerShape=Sphere  MarkerSize=10  GraphicVisPropType=SimpleVisualProperties  GraphicDiffuseColor=[1.0 0.4 0.4]  GraphicSpecularColor=[0.5 0.5 0.5 1.0]  GraphicAmbientColor=[0.15 0.15 0.15 1.0]  GraphicEmissiveColor=[0.0 0.0 0.0 1.0]  GraphicShininess=75  GraphicOpacity=smiData.Solid(5).opacity
  Transform : sm_lib/Frames and Transforms/Rigid Transform  TranslationMethod=Cartesian  TranslationStandardOffset=0  TranslationLengthUnit=mm  TranslationStandardAxis=+Z  TranslationCartesianOffset=smiData.RigidTransform(6).translation  TranslationROffset=0  TranslationROffsetUnits=m  TranslationZOffset=0  TranslationZOffsetUnits=m  TranslationThetaOffset=0  TranslationThetaOffsetUnits=deg  RotationMethod=ArbitraryAxis  RotationAngleUnits=rad  RotationStandardAxis=+Z  RotationAngle=smiData.RigidTransform(6).angle  RotationArbitraryAxis=smiData.RigidTransform(6).axis  FollAlignAxisA=+X  BaseAlignAxisA=+Y  FollAlignAxisB=+Y  BaseAlignAxisB=+Z  RotationSequenceAxes=FollowerAxes  RotationSequence=XYX  RotationSequenceAngles=[0 0 0]  RotationSequenceAnglesUnits=deg  RotationMatrix=[1 0 0; 0 1 0; 0 0 1]
  Transform1 : sm_lib/Frames and Transforms/Rigid Transform  TranslationMethod=Cartesian  TranslationStandardOffset=0  TranslationLengthUnit=mm  TranslationStandardAxis=+Z  TranslationCartesianOffset=smiData.RigidTransform(10).translation  TranslationROffset=0  TranslationROffsetUnits=m  TranslationZOffset=0  TranslationZOffsetUnits=m  TranslationThetaOffset=0  TranslationThetaOffsetUnits=deg  RotationMethod=ArbitraryAxis  RotationAngleUnits=rad  RotationStandardAxis=+Z  RotationAngle=smiData.RigidTransform(10).angle  RotationArbitraryAxis=smiData.RigidTransform(10).axis  FollAlignAxisA=+X  BaseAlignAxisA=+Y  FollAlignAxisB=+Y  BaseAlignAxisB=+Z  RotationSequenceAxes=FollowerAxes  RotationSequence=XYX  RotationSequenceAngles=[0 0 0]  RotationSequenceAnglesUnits=deg  RotationMatrix=[1 0 0; 0 1 0; 0 0 1]
  F1 : PMIOPort  Side=Left
  F : PMIOPort  Port=2  Side=Left
  connections:
  Solid/RConn1 -- ReferenceFrame/RConn1 -- Transform/LConn1 -- Transform1/LConn1
  Transform/RConn1 -- F/RConn1
  Transform1/RConn1 -- F1/RConn1

== system manipulator_identification_q3/Link 1/link_1c_base_1_RIGID ==
  ReferenceFrame : sm_lib/Frames and Transforms/Reference Frame
  Solid : sm_lib/Body Elements/File Solid  ExtGeomFileName=C:\Users\miche\OneDrive - unibs.it\University\Magistrale - UNIBS\1_Primo Anno\Servosystems & Robotics\Servosystems & Robotics Project\Robot Model - Solidworks\Manipulator\simscape_linked_assembly\link_1c_base_Default_sldprt.STEP  UnitType=FromFile  ExtGeomFileUnits=m  StepReaderType=HEX  ExportConvexHullGeometry=off  InertiaType=Custom  Mass=smiData.Solid(3).mass  MassUnits=kg  CenterOfMass=smiData.Solid(3).CoM  CenterOfMassUnits=cm  MomentsOfInertia=smiData.Solid(3).MoI  MomentsOfInertiaUnits=kg*cm^2  ProductsOfInertia=smiData.Solid(3).PoI  ProductsOfInertiaUnits=kg*cm^2  BasedOnType=DensityFromFile  Density=1000  DensityUnits=kg/m^3  DoExposeReferenceFrame=on  SerializedFrames=<Frames/>  GraphicType=FromGeometry  MarkerShape=Sphere  MarkerSize=10  GraphicVisPropType=SimpleVisualProperties  GraphicDiffuseColor=[1.0 0.4 0.4]  GraphicSpecularColor=[0.5 0.5 0.5 1.0]  GraphicAmbientColor=[0.15 0.15 0.15 1.0]  GraphicEmissiveColor=[0.0 0.0 0.0 1.0]  GraphicShininess=75  GraphicOpacity=smiData.Solid(3).opacity
  Transform : sm_lib/Frames and Transforms/Rigid Transform  TranslationMethod=Cartesian  TranslationStandardOffset=0  TranslationLengthUnit=mm  TranslationStandardAxis=+Z  TranslationCartesianOffset=smiData.RigidTransform(9).translation  TranslationROffset=0  TranslationROffsetUnits=m  TranslationZOffset=0  TranslationZOffsetUnits=m  TranslationThetaOffset=0  TranslationThetaOffsetUnits=deg  RotationMethod=ArbitraryAxis  RotationAngleUnits=rad  RotationStandardAxis=+Z  RotationAngle=smiData.RigidTransform(9).angle  RotationArbitraryAxis=smiData.RigidTransform(9).axis  FollAlignAxisA=+X  BaseAlignAxisA=+Y  FollAlignAxisB=+Y  BaseAlignAxisB=+Z  RotationSequenceAxes=FollowerAxes  RotationSequence=XYX  RotationSequenceAngles=[0 0 0]  RotationSequenceAnglesUnits=deg  RotationMatrix=[1 0 0; 0 1 0; 0 0 1]
  Transform1 : sm_lib/Frames and Transforms/Rigid Transform  TranslationMethod=Cartesian  TranslationStandardOffset=0  TranslationLengthUnit=mm  TranslationStandardAxis=+Z  TranslationCartesianOffset=smiData.RigidTransform(13).translation  TranslationROffset=0  TranslationROffsetUnits=m  TranslationZOffset=0  TranslationZOffsetUnits=m  TranslationThetaOffset=0  TranslationThetaOffsetUnits=deg  RotationMethod=ArbitraryAxis  RotationAngleUnits=rad  RotationStandardAxis=+Z  RotationAngle=smiData.RigidTransform(13).angle  RotationArbitraryAxis=smiData.RigidTransform(13).axis  FollAlignAxisA=+X  BaseAlignAxisA=+Y  FollAlignAxisB=+Y  BaseAlignAxisB=+Z  RotationSequenceAxes=FollowerAxes  RotationSequence=XYX  RotationSequenceAngles=[0 0 0]  RotationSequenceAnglesUnits=deg  RotationMatrix=[1 0 0; 0 1 0; 0 0 1]
  F1 : PMIOPort  Side=Left
  F : PMIOPort  Port=2  Side=Left
  connections:
  Solid/RConn1 -- ReferenceFrame/RConn1 -- Transform/LConn1 -- Transform1/LConn1
  Transform/RConn1 -- F/RConn1
  Transform1/RConn1 -- F1/RConn1
